simulink model "VehicleSteering_sim"  (R2020a)
settings: Solver=VariableStepAuto  StartTime=0.0  StopTime=10.0  RelTol=1e-3
values from neighbouring files (symbols this model uses):
  A = [0 v0;0 0]    [Example_VehicleSteering_Ackermann.m]    (also in Example_VehicleSteering_Integral_action.m = Ag; Example_VehicleSteering_SS_control.m)
  B = [a*v0/b v0/b]'    [Example_VehicleSteering_Ackermann.m]    (also in Example_VehicleSteering_Integral_action.m = Bg; Example_VehicleSteering_SS_control.m)
  C = eye(2)    [Example_VehicleSteering_Ackermann.m]    (also in Example_VehicleSteering_Integral_action.m = eye(3); Example_VehicleSteering_SS_control.m)
  D = [0 0]'    [Example_VehicleSteering_Ackermann.m]    (also in Example_VehicleSteering_Integral_action.m = [0 0 0]'; Example_VehicleSteering_SS_control.m)
  K = [p - ap] * Wr_tilde * Wr^(-1)    [Example_VehicleSteering_Ackermann.m]    (also in Example_VehicleSteering_Integral_action.m; Example_VehicleSteering_SS_control.m = [b*wn^2/v0^2 (2*zeta*wn*b/v0-a*b*wn^2/v0^2)])
  kr = -(C * (A1)^(-1) * B)^(-1)    [Example_VehicleSteering_Ackermann.m]    (also in Example_VehicleSteering_Integral_action.m = 1; Example_VehicleSteering_SS_control.m = 0.444444444444)
settings Model: Creator=jofr  LastModifiedBy=rodralez
settings DataIOCC: ReturnWorkspaceOutputs=off
settings DebuggingCC: ArithmeticOperatorsInVariantConditions=warning
settings SFSimCC: SimUseLocalCustomCode=off  CustomCodeUndefinedFunction=UseInterfaceOnly
settings RTWCC: RTWUseLocalCustomCode=off

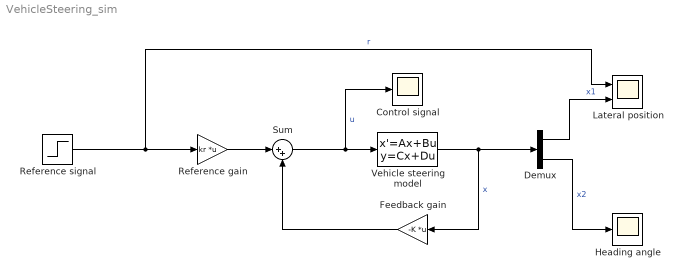
== system VehicleSteering_sim ==
  Control signal : Scope
  Demux : Demux  Outputs=2
  Feedback gain : Gain  Gain=-K  Multiplication=Matrix(K*u)
  Heading angle : Scope
  Lateral position : Scope  NumInputPorts=2
  Reference gain : Gain  Gain=kr  Multiplication=Matrix(K*u)
  "Reference signal " : Step  SampleTime=0
  Sum : Sum  Inputs=|++
  Vehicle steering model : StateSpace  A=A  B=B  C=C  D=D  InitialCondition=0
  wires:
  Vehicle steering model/1 -> Demux/1, Feedback gain/1  "x"
  Sum/1 -> Control signal/1, Vehicle steering model/1  "u"
  Feedback gain/1 -> Sum/2
  Reference gain/1 -> Sum/1
  Demux/2 -> Heading angle/1  "x2"
  "Reference signal "/1 -> Lateral position/1, Reference gain/1  "r"
  Demux/1 -> Lateral position/2  "x1"
